simulink model "inv_cart_pend_sf_control"  (R2018a)
settings: Solver=ode15s  StartTime=0.0  StopTime=5  RelTol=1e-3  EnableMultiTasking=on
settings Model: Creator=Arnab Banerjee  LastModifiedBy=Arnab Banerjee
settings DataIOCC: LimitDataPoints=on  SaveFormat=Array
settings OptimizationCC: LifeSpan=inf
settings DebuggingCC: SFUnexpectedBacktrackingDiag=warning  SFNoUnconditionalDefaultTransitionDiag=warning  SFExecutionAtInitializationDiag=none
settings HardwareCC: ProdBitPerPointer=32  ProdBitPerSizeT=32  ProdBitPerPtrDiffT=32  ProdLargestAtomicFloat=None  ProdIntDivRoundTo=Undefined  ProdEndianess=Unspecified  ProdWordSize=32  ProdHWDeviceType=32-bit Generic
settings ModelReferenceCC: PropagateSignalLabelsOutOfModel=off
settings CodeAppCC: StateflowObjectComments=on
settings GRTTargetCC: TargetLangStandard=C89/C90 (ANSI)  GeneratePreprocessorConditionals=Disable all
settings ConfigComp: CovMetricSettings=dw  CovHtmlReporting=on  CovSaveCumulativeToWorkspaceVar=on  CovSaveSingleToWorkspaceVar=on  CovExternalEMLEnable=off

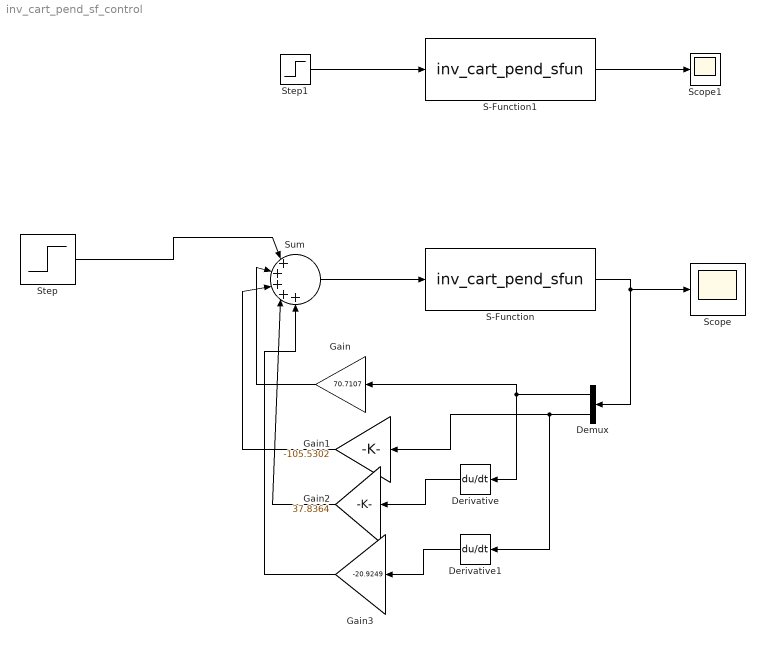
== system inv_cart_pend_sf_control ==
  Demux : Demux  Outputs=2
  Derivative : Derivative
  Derivative1 : Derivative
  Gain : Gain  Gain=70.7107
  Gain1 : Gain  Gain=-105.5302
  Gain2 : Gain  Gain=37.8364
  Gain3 : Gain  Gain=-20.9249
  S-Function : S-Function  FunctionName=inv_cart_pend_sfun  SFunctionDeploymentMode=off  EnableBusSupport=off
  S-Function1 : S-Function  FunctionName=inv_cart_pend_sfun  SFunctionDeploymentMode=off  EnableBusSupport=off
  Scope : Scope
  Scope1 : Scope
  Step : Step  Time=0  SampleTime=0
  Step1 : Step  Time=0  SampleTime=0
  Sum : Sum  Inputs=|+++++
  wires:
  S-Function/1 -> Demux/1, Scope/1
  Demux/1 -> Derivative/1, Gain/1
  Gain/1 -> Sum/2
  Demux/2 -> Derivative1/1, Gain1/1
  Gain1/1 -> Sum/3
  Derivative/1 -> Gain2/1
  Derivative1/1 -> Gain3/1
  Gain2/1 -> Sum/4
  Gain3/1 -> Sum/5
  Sum/1 -> S-Function/1
  S-Function1/1 -> Scope1/1
  Step/1 -> Sum/1
  Step1/1 -> S-Function1/1
